simulink model "Simulation"  (R2018b)
settings: Solver=VariableStepAuto  StartTime=0.0  StopTime=3  RelTol=1e-3
values from neighbouring files (symbols this model uses):
  Q = [0.01 0 ... (first row only)    [SimModelParams.m]    (also in runEKF.m)
  R = 0.5136    [SimModelParams.m]    (also in runEKF.m)
  SR_Lookup_Distance = [0 2 4 6 8 10 12 14 16 18 20 25 30 35 40]    [SimulationSection_Q1b.m]
  SR_Lookup_Voltage = [0 2.2 2.7 2 1.6 1.3 1.15 0.9 0.8 0.75 0.65 0.5 0.45 0.35 0.3]    [SimulationSection_Q1b.m]
  T = 0.5    [SimModelParams.m]    (also in runEKF.m = 0.1)
settings Model: Creator=Sachin  LastModifiedBy=sachin

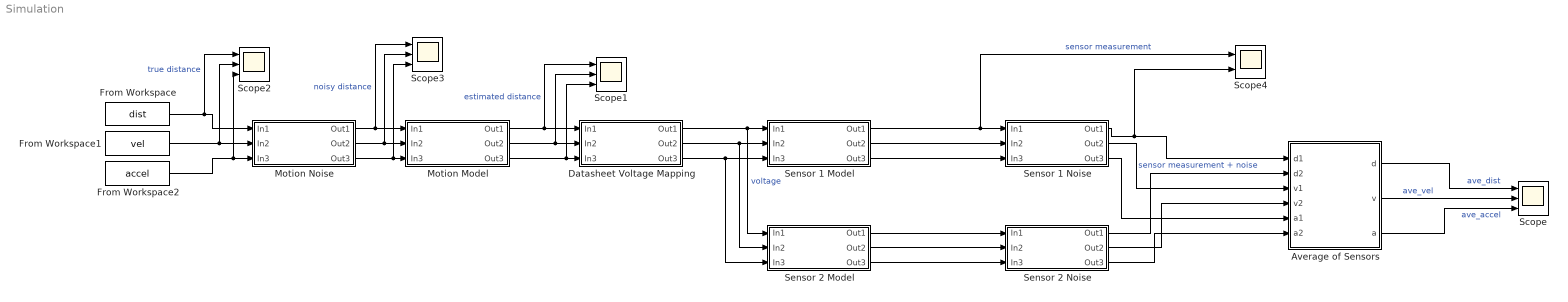
== system Simulation ==
  Average of Sensors : MATLAB Function  TreatAsAtomicUnit=on
  Datasheet Voltage Mapping : Subsystem
  From Workspace : FromWorkspace  VariableName=dist  SampleTime=0
  From Workspace1 : FromWorkspace  VariableName=vel  SampleTime=0
  From Workspace2 : FromWorkspace  VariableName=accel  SampleTime=0
  Motion Model : Subsystem
  Motion Noise : Subsystem
  Scope{,1..3} (4 alike) : Scope  NumInputPorts=3
  Scope4 : Scope  NumInputPorts=2
  Sensor 1 Model : Subsystem
  Sensor 1 Noise : Subsystem
  Sensor 2 Model : Subsystem
  Sensor 2 Noise : Subsystem
  wires:
  Motion Noise/1(Out1) -> Scope3/1, Motion Model/1(In1)  "noisy distance"
  Motion Noise/2(Out2) -> Scope3/2, Motion Model/2(In2)
  Motion Noise/3(Out3) -> Scope3/3, Motion Model/3(In3)
  Sensor 1 Model/1(Out1) -> Scope4/1, Sensor 1 Noise/1(In1)  "sensor measurement"
  Sensor 1 Model/2(Out2) -> Sensor 1 Noise/2(In2)
  Sensor 1 Model/3(Out3) -> Sensor 1 Noise/3(In3)
  Datasheet Voltage Mapping/1(Out1) -> Sensor 2 Model/1(In1), Sensor 1 Model/1(In1)  "voltage"
  Datasheet Voltage Mapping/2(Out2) -> Sensor 2 Model/2(In2), Sensor 1 Model/2(In2)
  Sensor 2 Model/3(Out3) -> Sensor 2 Noise/3(In3)
  Datasheet Voltage Mapping/3(Out3) -> Sensor 2 Model/3(In3), Sensor 1 Model/3(In3)
  Sensor 2 Model/1(Out1) -> Sensor 2 Noise/1(In1)
  Sensor 2 Model/2(Out2) -> Sensor 2 Noise/2(In2)
  Sensor 1 Noise/1(Out1) -> Scope4/2, Average of Sensors/1(d1)  "sensor measurement + noise"
  Sensor 2 Noise/1(Out1) -> Average of Sensors/2(d2)
  Sensor 1 Noise/2(Out2) -> Average of Sensors/3(v1)
  Sensor 2 Noise/2(Out2) -> Average of Sensors/4(v2)
  Sensor 1 Noise/3(Out3) -> Average of Sensors/5(a1)
  Sensor 2 Noise/3(Out3) -> Average of Sensors/6(a2)
  Motion Model/1(Out1) -> Scope1/1, Datasheet Voltage Mapping/1(In1)  "estimated distance"
  Motion Model/2(Out2) -> Scope1/2, Datasheet Voltage Mapping/2(In2)
  Motion Model/3(Out3) -> Scope1/3, Datasheet Voltage Mapping/3(In3)
  Average of Sensors/1(d) -> Scope/1  "ave_dist"
  Average of Sensors/2(v) -> Scope/2  "ave_vel"
  Average of Sensors/3(a) -> Scope/3  "ave_accel"
  From Workspace/1 -> Scope2/1, Motion Noise/1(In1)  "true distance"
  From Workspace1/1 -> Scope2/2, Motion Noise/2(In2)
  From Workspace2/1 -> Scope2/3, Motion Noise/3(In3)

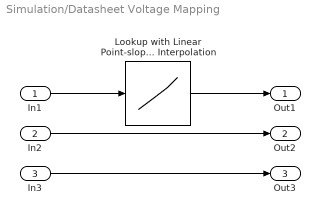
== system Simulation/Datasheet Voltage Mapping ==
  In1 : Inport
  In2 : Inport  Port=2
  In3 : Inport  Port=3
  Lookup with Linear Point-slope Interpolation : Lookup_n-D  NumberOfTableDimensions=1  BreakpointsForDimension1=SR_Lookup_Distance  Table=SR_Lookup_Voltage  InternalRulePriority=Speed  RndMeth=Simplest  InputSameDT=on
  Out1 : Outport
  Out2 : Outport  Port=2
  Out3 : Outport  Port=3
  wires:
  In2/1 -> Out2/1
  In3/1 -> Out3/1
  In1/1 -> Lookup with Linear Point-slope Interpolation/1
  Lookup with Linear Point-slope Interpolation/1 -> Out1/1

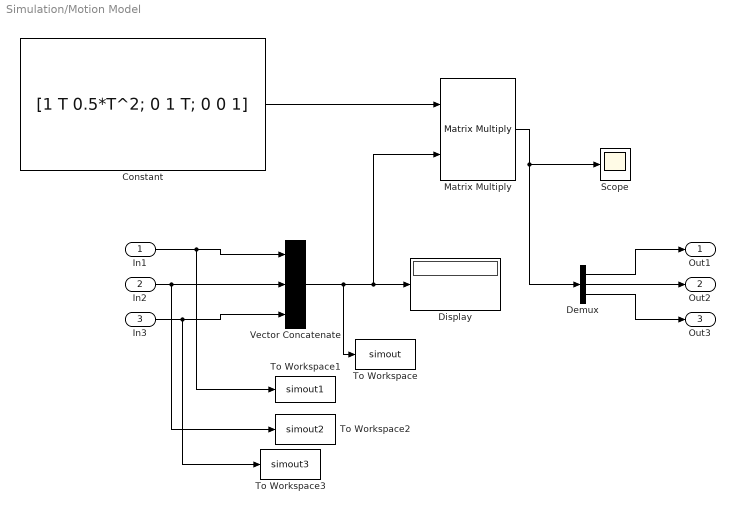
== system Simulation/Motion Model ==
  In1 : Inport
  In2 : Inport  Port=2
  In3 : Inport  Port=3
  Constant : Constant  Value=[1 T 0.5*T^2; 0 1 T; 0 0 1]  VectorParams1D=off
  Demux : Demux  Outputs=3
  Display : Display
  Matrix Multiply : Product  Multiplication=Matrix(*)
  Scope : Scope
  To Workspace : ToWorkspace  VariableName=simout  SaveFormat=Timeseries  SampleTime=-1
  To Workspace1 : ToWorkspace  VariableName=simout1  SaveFormat=Timeseries  SampleTime=-1
  To Workspace2 : ToWorkspace  VariableName=simout2  SaveFormat=Timeseries  SampleTime=-1
  To Workspace3 : ToWorkspace  VariableName=simout3  SaveFormat=Timeseries  SampleTime=-1
  Vector Concatenate : Concatenate  NumInputs=3
  Out1 : Outport
  Out2 : Outport  Port=2
  Out3 : Outport  Port=3
  wires:
  Constant/1 -> Matrix Multiply/1
  Vector Concatenate/1 -> To Workspace/1, Matrix Multiply/2, Display/1
  Matrix Multiply/1 -> Scope/1, Demux/1
  Demux/1 -> Out1/1
  Demux/2 -> Out2/1
  Demux/3 -> Out3/1
  In1/1 -> To Workspace1/1, Vector Concatenate/1
  In2/1 -> To Workspace2/1, Vector Concatenate/2
  In3/1 -> To Workspace3/1, Vector Concatenate/3

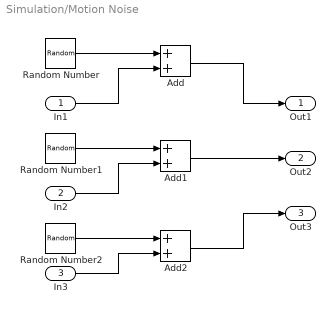
== system Simulation/Motion Noise ==
  In1 : Inport
  In2 : Inport  Port=2
  In3 : Inport  Port=3
  Add : Sum
  Add1 : Sum
  Add2 : Sum
  Random Number : RandomNumber  Variance=Q(1,1)  SampleTime=T
  Random Number1 : RandomNumber  Variance=Q(2, 2)  SampleTime=T
  Random Number2 : RandomNumber  Variance=Q(3,3)  SampleTime=T
  Out1 : Outport
  Out2 : Outport  Port=2
  Out3 : Outport  Port=3
  wires:
  In1/1 -> Add/2
  In2/1 -> Add1/2
  In3/1 -> Add2/2
  Random Number/1 -> Add/1
  Add/1 -> Out1/1
  Random Number1/1 -> Add1/1
  Add1/1 -> Out2/1
  Random Number2/1 -> Add2/1
  Add2/1 -> Out3/1

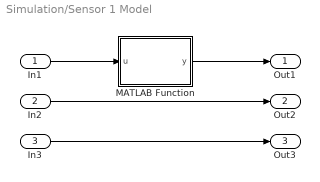
== system Simulation/Sensor 1 Model ==
  In1 : Inport
  In2 : Inport  Port=2
  In3 : Inport  Port=3
  MATLAB Function : MATLAB Function  TreatAsAtomicUnit=on
  Out1 : Outport
  Out2 : Outport  Port=2
  Out3 : Outport  Port=3
  wires:
  In1/1 -> MATLAB Function/1(u)
  In2/1 -> Out2/1
  In3/1 -> Out3/1
  MATLAB Function/1(y) -> Out1/1

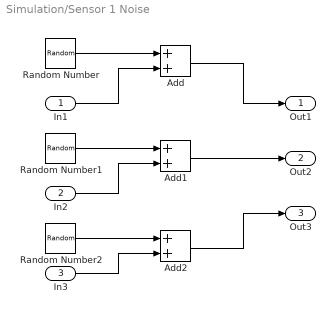
== system Simulation/Sensor 1 Noise ==
  In1 : Inport
  In2 : Inport  Port=2
  In3 : Inport  Port=3
  Add : Sum
  Add1 : Sum
  Add2 : Sum
  Random Number : RandomNumber  Variance=R(1)  SampleTime=T
  Random Number1 : RandomNumber  Variance=R(2)  SampleTime=T
  Random Number2 : RandomNumber  Variance=R(3)  SampleTime=T
  Out1 : Outport
  Out2 : Outport  Port=2
  Out3 : Outport  Port=3
  wires:
  In1/1 -> Add/2
  In2/1 -> Add1/2
  In3/1 -> Add2/2
  Random Number/1 -> Add/1
  Add/1 -> Out1/1
  Random Number1/1 -> Add1/1
  Add1/1 -> Out2/1
  Random Number2/1 -> Add2/1
  Add2/1 -> Out3/1

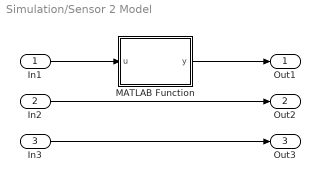
== system Simulation/Sensor 2 Model ==
  In1 : Inport
  In2 : Inport  Port=2
  In3 : Inport  Port=3
  MATLAB Function : MATLAB Function  TreatAsAtomicUnit=on
  Out1 : Outport
  Out2 : Outport  Port=2
  Out3 : Outport  Port=3
  wires:
  In1/1 -> MATLAB Function/1(u)
  In2/1 -> Out2/1
  In3/1 -> Out3/1
  MATLAB Function/1(y) -> Out1/1

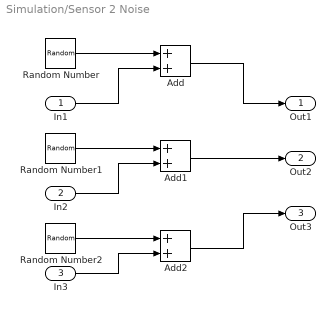
== system Simulation/Sensor 2 Noise ==
  In1 : Inport
  In2 : Inport  Port=2
  In3 : Inport  Port=3
  Add : Sum
  Add1 : Sum
  Add2 : Sum
  Random Number : RandomNumber  Variance=R(1)  SampleTime=T
  Random Number1 : RandomNumber  Variance=R(2)  SampleTime=T
  Random Number2 : RandomNumber  Variance=R(3)  SampleTime=T
  Out1 : Outport
  Out2 : Outport  Port=2
  Out3 : Outport  Port=3
  wires:
  In1/1 -> Add/2
  In2/1 -> Add1/2
  In3/1 -> Add2/2
  Random Number/1 -> Add/1
  Add/1 -> Out1/1
  Random Number1/1 -> Add1/1
  Add1/1 -> Out2/1
  Random Number2/1 -> Add2/1
  Add2/1 -> Out3/1

== matlab function Simulation/Sensor 2 Model/MATLAB Function ==
  data: u input; y output
function y = fcn(u)

X = 5.224514.^5113 / ((u+2.468841).^5113);

y = nthroot(X, 1014) + 2.196009;

== matlab function Simulation/Sensor 1 Model/MATLAB Function ==
  data: u input; y output
function y = fcn(u)
A = 5.224514;
B = -2.196009;
C = 0.198318;
D = -2.468841;

y = (((u - D) / A)^(-1/C)) - B;

== matlab function Simulation/Average of Sensors ==
  data: d1 input; d output; d2 input; v1 input; v2 input; a1 input; a2 input; v output; a output
function [d, v, a] = fcn(d1, d2, v1, v2, a1, a2)

d = (d1 + d2) / 2;
v = (v1 + v2) / 2;
a = (a1 + a2) / 2;
